simulink model "PruebaSupervisoryLogic"  (R2022a)
settings: Solver=VariableStepAuto  StartTime=0.0  StopTime=100  RelTol=1e-3
values from neighbouring files (symbols this model uses):
  a = 0.2    [Data.m]
  alturaobst = 0.9    [Data.m]
  b = 0.542    [Data.m]
  M = [x_new y_new]    [Data.m]
  M_chasis = 3.5    [Data.m]
  M_rueda = 1    [Data.m]
  M_ruedacontacto = 1    [Data.m]
  N = 4365    [GraficasVelocidades.m]    (also in Prueba_Liapunov.m = length(p_X); WaypointsToTrayectory.m = length(X))
  R = 0.175/2    (= 0.0875)    [Data.m]
  X = M(:,1)    [WaypointsToTrayectory.m]
  x0 = x_ini(1)*factorE    [Data.m]
  x_obj = pos_fin(1)*factorE    [Data.m]
  xobstac = RandomPos(1)    [Data.m]
  Y = M(:, 2)    [WaypointsToTrayectory.m]
  y0 = y_ini(2)*factorE    [Data.m]
  y_obj = pos_fin(2)*factorE    [Data.m]
  yobstac = RandomPos(2)    [Data.m]
  zobstac = RandomPos(3)    [Data.m]
undefined symbols (not defined in the file or in its folder): bloqueobstaculo, Borde11, Borde12, Borde2, Borde3, Borde41, Borde42, Explanada, plano150g1, plano150g2, plano150g3, plano150g4, Plano150mm, plano150mm2irr, Plano45mm, plano45mm2irr, Plano90mm, Rampa, Rampa21, Rampa22, Rampa31, Rampa32, Rampa33, Rampa4, Rampa51, Rampa52, Rampa53, Terreno, Z
libraries: sm_lib x331, nesl_utility x30, fl_lib x3, robotalgslib x1
(part 2 of 8)

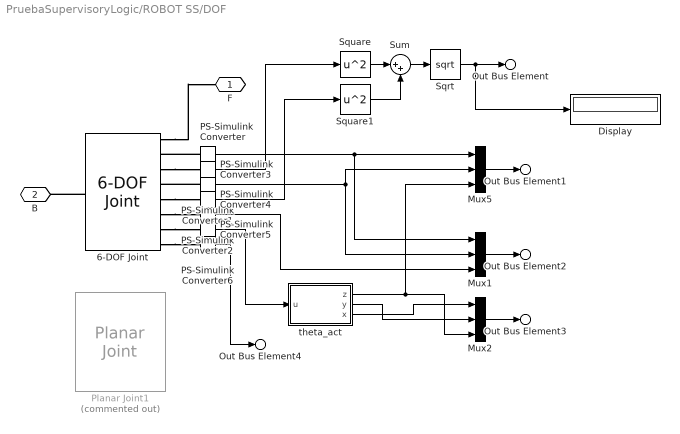
== system PruebaSupervisoryLogic/ROBOT SS/DOF ==
  6-DOF Joint : sm_lib/Joints/6-DOF Joint  JointMode=Normal  SenseConstraintForce=off  SenseConstraintForceX=off  SenseConstraintForceY=off  SenseConstraintForceZ=off  SenseConstraintTorque=off  SenseConstraintTorqueX=off  SenseConstraintTorqueY=off  SenseConstraintTorqueZ=off  SenseTotalForce=off  SenseTotalForceX=off  SenseTotalForceY=off  SenseTotalForceZ=off  SenseTotalTorque=off  SenseTotalTorqueX=off  SenseTotalTorqueY=off  SenseTotalTorqueZ=off  CompositeWrenchDir=FollowerOnBase  CompositeWrenchFrame=BaseFrame  PxEquilibriumPosition=0  PxEquilibriumPositionUnits=m  PxSpringStiffness=0  PxSpringStiffnessUnits=N/m  PxDampingCoefficient=0  PxDampingCoefficientUnits=N/(m/s)  PxTorqueActuationMode=NoTorque  PxMotionActuationMode=ComputedMotion  PxSensePosition=on  PxSenseVelocity=on  PxSenseAcceleration=off  PxSenseTorqueForce=off  PxSenseLowerLimitTorqueForce=off  PxSenseUpperLimitTorqueForce=off  PxLowerLimitSpecify=off  PxLowerLimitBound=-1  PxLowerLimitBoundUnits=m  PxLowerLimitStiffness=1e6  PxLowerLimitStiffnessUnits=N/m  PxLowerLimitDamping=1e3  PxLowerLimitDampingUnits=N/(m/s)  PxLowerLimitTransitionRegionWidth=1e-4  PxLowerLimitTransitionRegionWidthUnits=m  PxUpperLimitSpecify=off  PxUpperLimitBound=1  PxUpperLimitBoundUnits=m  PxUpperLimitStiffness=1e6  PxUpperLimitStiffnessUnits=N/m  PxUpperLimitDamping=1e3  PxUpperLimitDampingUnits=N/(m/s)  PxUpperLimitTransitionRegionWidth=1e-4  PxUpperLimitTransitionRegionWidthUnits=m  PxPositionTargetSpecify=on  PxPositionTargetPriority=High  PxPositionTargetValue=x0  PxPositionTargetValueUnits=m  PxVelocityTargetSpecify=off  PxVelocityTargetPriority=High  PxVelocityTargetValue=0  PxVelocityTargetValueUnits=m/s  PyEquilibriumPosition=0  PyEquilibriumPositionUnits=m  PySpringStiffness=0  PySpringStiffnessUnits=N/m  PyDampingCoefficient=0  PyDampingCoefficientUnits=N/(m/s)  PyTorqueActuationMode=NoTorque  PyMotionActuationMode=ComputedMotion  PySensePosition=on  PySenseVelocity=on  PySenseAcceleration=off  PySenseTorqueForce=off  PySenseLowerLimitTorqueForce=off  PySenseUpperLimitTorqueForce=off  PyLowerLimitSpecify=off  PyLowerLimitBound=-1  PyLowerLimitBoundUnits=m  PyLowerLimitStiffness=1e6  PyLowerLimitStiffnessUnits=N/m  PyLowerLimitDamping=1e3  PyLowerLimitDampingUnits=N/(m/s)  PyLowerLimitTransitionRegionWidth=1e-4  PyLowerLimitTransitionRegionWidthUnits=m  PyUpperLimitSpecify=off  PyUpperLimitBound=1  PyUpperLimitBoundUnits=m  PyUpperLimitStiffness=1e6  PyUpperLimitStiffnessUnits=N/m  PyUpperLimitDamping=1e3  PyUpperLimitDampingUnits=N/(m/s)  PyUpperLimitTransitionRegionWidth=1e-4  PyUpperLimitTransitionRegionWidthUnits=m  PyPositionTargetSpecify=on  PyPositionTargetPriority=High  PyPositionTargetValue=y0  PyPositionTargetValueUnits=m  PyVelocityTargetSpecify=off  PyVelocityTargetPriority=High  PyVelocityTargetValue=0  PyVelocityTargetValueUnits=m/s  PzEquilibriumPosition=0  PzEquilibriumPositionUnits=m  PzSpringStiffness=0  PzSpringStiffnessUnits=N/m  PzDampingCoefficient=0  PzDampingCoefficientUnits=N/(m/s)  PzTorqueActuationMode=NoTorque  PzMotionActuationMode=ComputedMotion  PzSensePosition=on  PzSenseVelocity=off  PzSenseAcceleration=off  PzSenseTorqueForce=off  PzSenseLowerLimitTorqueForce=off  PzSenseUpperLimitTorqueForce=off  PzLowerLimitSpecify=off  PzLowerLimitBound=-1  PzLowerLimitBoundUnits=m  PzLowerLimitStiffness=1e6  PzLowerLimitStiffnessUnits=N/m  PzLowerLimitDamping=1e3  PzLowerLimitDampingUnits=N/(m/s)  PzLowerLimitTransitionRegionWidth=1e-4  PzLowerLimitTransitionRegionWidthUnits=m  PzUpperLimitSpecify=off  PzUpperLimitBound=1  PzUpperLimitBoundUnits=m  PzUpperLimitStiffness=1e6  PzUpperLimitStiffnessUnits=N/m  PzUpperLimitDamping=1e3  PzUpperLimitDampingUnits=N/(m/s)  PzUpperLimitTransitionRegionWidth=1e-4  PzUpperLimitTransitionRegionWidthUnits=m  PzPositionTargetSpecify=off  PzPositionTargetPriority=High  PzPositionTargetValue=1  PzPositionTargetValueUnits=m  PzVelocityTargetSpecify=off  PzVelocityTargetPriority=High  PzVelocityTargetValue=0  PzVelocityTargetValueUnits=m/s  SphDefPosRotationMethod=None  SphDefPosRotationAngleUnits=deg  SphDefPosRotationStandardAxis=+Z  SphDefPosRotationAngle=0.0  SphDefPosRotationArbitraryAxis=[0 0 1]  SphDefPosFollAlignAxisA=+X  SphDefPosBaseAlignAxisA=+Y  SphDefPosFollAlignAxisB=+Y  SphDefPosBaseAlignAxisB=+Z  SphDefPosRotationSequenceAxes=FollowerAxes  SphDefPosRotationSequence=XYX  SphDefPosRotationSequenceAngles=[0 0 0]  SphDefPosRotationSequenceAnglesUnits=deg  SphDefPosRotationMatrix=[1 0 0; 0 1 0; 0 0 1]  SphEqPosRotationMethod=None  SphEqPosRotationAngleUnits=deg  SphEqPosRotationStandardAxis=+Z  SphEqPosRotationAngle=0.0  SphEqPosRotationArbitraryAxis=[0 0 1]  SphEqPosFollAlignAxisA=+X  SphEqPosBaseAlignAxisA=+Y  SphEqPosFollAlignAxisB=+Y  SphEqPosBaseAlignAxisB=+Z  SphEqPosRotationSequenceAxes=FollowerAxes  SphEqPosRotationSequence=XYX  SphEqPosRotationSequenceAngles=[0 0 0]  SphEqPosRotationSequenceAnglesUnits=deg  SphEqPosRotationMatrix=[1 0 0; 0 1 0; 0 0 1]  SphSpringStiffness=0  SphSpringStiffnessUnits=N*m/deg  SphDampingCoefficient=0  SphDampingCoefficientUnits=N*m/(deg/s)  SphActuateTorqueX=off  SphActuateTorqueY=off  SphActuateTorqueZ=off  SphActuateTorque=off  SphTorqueActuationMode=NoTorque  SphMotionActuationMode=ComputedMotion  SphActuationFrame=BaseFrame  SphSensePosition=on  SphSenseVelocityX=off  SphSenseVelocityY=off  SphSenseVelocityZ=on  SphSenseVelocity=off  SphSenseAccelerationX=off  SphSenseAccelerationY=off  SphSenseAccelerationZ=off  SphSenseAcceleration=off  SphSenseTorqueX=off  SphSenseTorqueY=off  SphSenseTorqueZ=off  SphSenseTorqueForce=off  SphSenseLowerLimitTorqueMag=off  SphSenseUpperLimitTorqueMag=off  SphSensingFrame=BaseFrame  SphLowerLimitSpecify=off  SphLowerLimitBound=15  SphLowerLimitBoundUnits=deg  SphLowerLimitStiffness=1e4  SphLowerLimitStiffnessUnits=N*m/deg  SphLowerLimitDamping=10  SphLowerLimitDampingUnits=N*m/(deg/s)  SphLowerLimitTransitionRegionWidth=0.1  SphLowerLimitTransitionRegionWidthUnits=deg  SphUpperLimitSpecify=off  SphUpperLimitBound=45  SphUpperLimitBoundUnits=deg  SphUpperLimitStiffness=1e4  SphUpperLimitStiffnessUnits=N*m/deg  SphUpperLimitDamping=10  SphUpperLimitDampingUnits=N*m/(deg/s)  SphUpperLimitTransitionRegionWidth=0.1  SphUpperLimitTransitionRegionWidthUnits=deg  SphPositionTargetRotationMethod=StandardAxis  SphPositionTargetRotationAngleUnits=rad  SphPositionTargetRotationStandardAxis=+Z  SphPositionTargetRotationAngle=2*pi  SphPositionTargetRotationArbitraryAxis=[0 0 1]  SphPositionTargetFollAlignAxisA=+X  SphPositionTargetBaseAlignAxisA=+Y  SphPositionTargetFollAlignAxisB=+Y  SphPositionTargetBaseAlignAxisB=+Z  SphPositionTargetRotationSequenceAxes=FollowerAxes  SphPositionTargetRotationSequence=ZYX  SphPositionTargetRotationSequenceAngles=[0.0532 -0.048 0.0147]  SphPositionTargetRotationSequenceAnglesUnits=rad  SphPositionTargetRotationMatrix=[1 0 0; 0 1 0; 0 0 1]  SphPositionTargetSpecify=on  SphPositionTargetPriority=High  SphVelocityTargetValue=[0 0 0]  SphVelocityTargetValueUnits=deg/s  SphVelocityTargetSpecify=off  SphVelocityTargetPriority=High  SphVelocityTargetInFollowerFrame=on
  Display : Display
  Mux1 : Mux  Inputs=3
  Mux2 : Mux  Inputs=3
  Mux5 : Mux  Inputs=3
  PS-Simulink Converter{,1..6} (7 alike) : nesl_utility/PS-Simulink Converter  PhysicalDomain=network_engine_domain  SubClassName=ps_output  LeftPortType=input  RightPortType=output  PseudoPeriodic=off  Frequencies=[]  VectorFormat=inherit  Unit=inherit  AffineConversion=off
      settings: SourceProductBaseCode=SS,PW,VE
  Planar Joint1 : sm_lib/Joints/Planar Joint  Commented=on  JointMode=Normal  SenseConstraintForce=off  SenseConstraintForceX=off  SenseConstraintForceY=off  SenseConstraintForceZ=off  SenseConstraintTorque=off  SenseConstraintTorqueX=off  SenseConstraintTorqueY=off  SenseConstraintTorqueZ=off  SenseTotalForce=off  SenseTotalForceX=off  SenseTotalForceY=off  SenseTotalForceZ=off  SenseTotalTorque=off  SenseTotalTorqueX=off  SenseTotalTorqueY=off  SenseTotalTorqueZ=off  CompositeWrenchDir=FollowerOnBase  CompositeWrenchFrame=BaseFrame  PxEquilibriumPosition=0  PxEquilibriumPositionUnits=m  PxSpringStiffness=0  PxSpringStiffnessUnits=N/m  PxDampingCoefficient=0  PxDampingCoefficientUnits=N/(m/s)  PxTorqueActuationMode=NoTorque  PxMotionActuationMode=ComputedMotion  PxSensePosition=on  PxSenseVelocity=off  PxSenseAcceleration=off  PxSenseTorqueForce=off  PxSenseLowerLimitTorqueForce=off  PxSenseUpperLimitTorqueForce=off  PxLowerLimitSpecify=off  PxLowerLimitBound=-1  PxLowerLimitBoundUnits=m  PxLowerLimitStiffness=1e6  PxLowerLimitStiffnessUnits=N/m  PxLowerLimitDamping=1e3  PxLowerLimitDampingUnits=N/(m/s)  PxLowerLimitTransitionRegionWidth=1e-4  PxLowerLimitTransitionRegionWidthUnits=m  PxUpperLimitSpecify=off  PxUpperLimitBound=1  PxUpperLimitBoundUnits=m  PxUpperLimitStiffness=1e6  PxUpperLimitStiffnessUnits=N/m  PxUpperLimitDamping=1e3  PxUpperLimitDampingUnits=N/(m/s)  PxUpperLimitTransitionRegionWidth=1e-4  PxUpperLimitTransitionRegionWidthUnits=m  PxPositionTargetSpecify=on  PxPositionTargetPriority=High  PxPositionTargetValue=540  PxPositionTargetValueUnits=m  PxVelocityTargetSpecify=off  PxVelocityTargetPriority=High  PxVelocityTargetValue=0  PxVelocityTargetValueUnits=m/s  PyEquilibriumPosition=0  PyEquilibriumPositionUnits=m  PySpringStiffness=0  PySpringStiffnessUnits=N/m  PyDampingCoefficient=0  PyDampingCoefficientUnits=N/(m/s)  PyTorqueActuationMode=NoTorque  PyMotionActuationMode=ComputedMotion  PySensePosition=on  PySenseVelocity=off  PySenseAcceleration=off  PySenseTorqueForce=off  PySenseLowerLimitTorqueForce=off  PySenseUpperLimitTorqueForce=off  PyLowerLimitSpecify=off  PyLowerLimitBound=-1  PyLowerLimitBoundUnits=m  PyLowerLimitStiffness=1e6  PyLowerLimitStiffnessUnits=N/m  PyLowerLimitDamping=1e3  PyLowerLimitDampingUnits=N/(m/s)  PyLowerLimitTransitionRegionWidth=1e-4  PyLowerLimitTransitionRegionWidthUnits=m  PyUpperLimitSpecify=off  PyUpperLimitBound=1  PyUpperLimitBoundUnits=m  PyUpperLimitStiffness=1e6  PyUpperLimitStiffnessUnits=N/m  PyUpperLimitDamping=1e3  PyUpperLimitDampingUnits=N/(m/s)  PyUpperLimitTransitionRegionWidth=1e-4  PyUpperLimitTransitionRegionWidthUnits=m  PyPositionTargetSpecify=on  PyPositionTargetPriority=High  PyPositionTargetValue=241  PyPositionTargetValueUnits=m  PyVelocityTargetSpecify=off  PyVelocityTargetPriority=High  PyVelocityTargetValue=0  PyVelocityTargetValueUnits=m/s  RzEquilibriumPosition=0  RzEquilibriumPositionUnits=deg  RzSpringStiffness=0  RzSpringStiffnessUnits=N*m/deg  RzDampingCoefficient=0  RzDampingCoefficientUnits=N*m/(deg/s)  RzTorqueActuationMode=NoTorque  RzMotionActuationMode=ComputedMotion  RzSensePosition=on  RzSenseVelocity=off  RzSenseAcceleration=off  RzSenseTorqueForce=off  RzSenseLowerLimitTorqueForce=off  RzSenseUpperLimitTorqueForce=off  RzLowerLimitSpecify=off  RzLowerLimitBound=-90  RzLowerLimitBoundUnits=deg  RzLowerLimitStiffness=1e4  RzLowerLimitStiffnessUnits=N*m/deg  RzLowerLimitDamping=10  RzLowerLimitDampingUnits=N*m/(deg/s)  RzLowerLimitTransitionRegionWidth=0.1  RzLowerLimitTransitionRegionWidthUnits=deg  RzUpperLimitSpecify=off  RzUpperLimitBound=90  RzUpperLimitBoundUnits=deg  RzUpperLimitStiffness=1e4  RzUpperLimitStiffnessUnits=N*m/deg  RzUpperLimitDamping=10  RzUpperLimitDampingUnits=N*m/(deg/s)  RzUpperLimitTransitionRegionWidth=0.1  RzUpperLimitTransitionRegionWidthUnits=deg  RzPositionTargetSpecify=on  RzPositionTargetPriority=High  RzPositionTargetValue=2*pi/3  RzPositionTargetValueUnits=rad  RzVelocityTargetSpecify=off  RzVelocityTargetPriority=High  RzVelocityTargetValue=0  RzVelocityTargetValueUnits=deg/s
  Sqrt : Sqrt
  Square : Math  Operator=square
  Square1 : Math  Operator=square
  Sum : Sum  Inputs=|++
  theta_act : MATLAB Function  TreatAsAtomicUnit=on
  F : PMIOPort  Side=Right
  B : PMIOPort  Port=2  Side=Left
  Out Bus Element : Outport  PortName=dof  Element=v
  Out Bus Element1 : Outport  PortName=dof  Element=Pose
  Out Bus Element2 : Outport  PortName=dof  Element=xyz
  Out Bus Element3 : Outport  PortName=dof  Element=rpy
  Out Bus Element4 : Outport  PortName=dof  Element=wz
  wires:
  PS-Simulink Converter/1 -> Mux1/1, Mux5/1
  Mux5/1 -> Out Bus Element1/1
  PS-Simulink Converter1/1 -> Mux1/2, Mux5/2
  Square1/1 -> Sum/2
  PS-Simulink Converter4/1 -> Square1/1
  Sum/1 -> Sqrt/1
  Square/1 -> Sum/1
  PS-Simulink Converter3/1 -> Square/1
  Sqrt/1 -> Display/1, Out Bus Element/1
  PS-Simulink Converter2/1 -> Mux1/3
  Mux1/1 -> Out Bus Element2/1
  PS-Simulink Converter5/1 -> theta_act/1(u)
  theta_act/1(z) -> Mux5/3, Mux2/3
  theta_act/3(x) -> Mux2/1
  theta_act/2(y) -> Mux2/2
  Mux2/1 -> Out Bus Element3/1
  PS-Simulink Converter6/1 -> Out Bus Element4/1
  connections:
  PS-Simulink Converter/LConn1 -- 6-DOF Joint/RConn2
  6-DOF Joint/LConn1 -- B/RConn1
  PS-Simulink Converter1/LConn1 -- 6-DOF Joint/RConn4
  6-DOF Joint/RConn1 -- F/RConn1
  6-DOF Joint/RConn3 -- PS-Simulink Converter3/LConn1
  6-DOF Joint/RConn5 -- PS-Simulink Converter4/LConn1
  6-DOF Joint/RConn6 -- PS-Simulink Converter2/LConn1
  6-DOF Joint/RConn7 -- PS-Simulink Converter5/LConn1
  6-DOF Joint/RConn8 -- PS-Simulink Converter6/LConn1

== system PruebaSupervisoryLogic/ROBOT SS/DesPathViz ==
  Desired Path Viz : sm_lib/Curves and Surfaces/Point Cloud  CoordinatesMatrix=pointCloud  CoordinatesMatrixUnits=m  GraphicType=MarkerCloud  GraphicSphereRadius=0.03  GraphicSphereRadiusUnits=m  GraphicVisPropType=SimpleVisualProperties  GraphicDiffuseColor=[0 0 1]  GraphicOpacity=1  GraphicSpecularColor=[0.5 0.5 0.5 1.0]  GraphicAmbientColor=[0.15 0.15 0.15 1.0]  GraphicEmissiveColor=[0.0 0.0 0.0 1.0]  GraphicShininess=75
      settings: SourceProductBaseCode=MS
  Rigid Transform6 : sm_lib/Frames and Transforms/Rigid Transform  TranslationMethod=Cartesian  TranslationStandardOffset=1.85  TranslationLengthUnit=m  TranslationStandardAxis=+Z  TranslationCartesianOffset=[0 0 0]  TranslationROffset=0  TranslationROffsetUnits=m  TranslationZOffset=0  TranslationZOffsetUnits=m  TranslationThetaOffset=0  TranslationThetaOffsetUnits=deg  RotationMethod=None  RotationAngleUnits=deg  RotationStandardAxis=+X  RotationAngle=90  RotationArbitraryAxis=[0 0 1]  FollAlignAxisA=+X  BaseAlignAxisA=+Y  FollAlignAxisB=+Y  BaseAlignAxisB=+Z  RotationSequenceAxes=FollowerAxes  RotationSequence=XYX  RotationSequenceAngles=[0 0 0]  RotationSequenceAnglesUnits=deg  RotationMatrix=[1 0 0; 0 1 0; 0 0 1]
  Spline : sm_lib/Curves and Surfaces/Spline  GraphicAmbientColor=[0.15 0.15 0.15 1.0]  GraphicDiffuseColor=[0 0.4471 0.7412]  DataPoints=pointCloud  DataPointsUnits=m  GraphicEmissiveColor=[0.0 0.0 0.0 1.0]  EndConditionType=Natural  MarkerShape=Sphere  MarkerSize=10  GraphicType=FromGeometry  GraphicOpacity=1  GraphicShininess=75  GraphicSpecularColor=[0.5 0.5 0.5 1.0]  GraphicVisPropType=SimpleVisualProperties
  R : PMIOPort  Side=Left
  connections:
  R/RConn1 -- Rigid Transform6/LConn1
  Rigid Transform6/RConn1 -- Desired Path Viz/LConn1 -- Spline/LConn1

== system PruebaSupervisoryLogic/ROBOT SS/Ensamble robot ==
  In1 : Inport
  In2 : Inport  Port=2
  Chasis : Subsystem
      settings: PortSchema="{\"entries\":[{\"content\":{\"sides\":[{\"content\":{\"connectorIds\":[\"LConn1\",\"LConn2\"]},\"type\":\"ConnectorPlacement.EquallySpacedRectSide\",\"uuid\":\"70add61d-4d2b-4209-9064-ae93618a5dda\"},{\"content\":{\"connectorIds\":[\"RConn1\",\"RConn2\"],\"side\":\"RIGHT\"},\"type\":\"ConnectorPlacement.EquallySpacedRectSide\",\"uuid\":\"c0cb1301-4b60-4f09-9729-118a381e7d2b\"},{\"content\":{\"connectorIds\":[\"LConn3\",\"LConn4\"],\"side\":\"TOP\"},\"type\":\"ConnectorPlacement.EquallySpacedRectSide\",\"uuid\":\"bcc4c9f8-927c-42da-82df-989f649289ae\"},{\"content\":{\"connectorIds\":[\"RConn3\"],\"side\":\"BOTTOM\"},\"type\":\"ConnectorPlacement.EquallySpacedRectSide\",\"uuid\":\"275f36ca-265b-4208-becd-8d42af8e2e6a\"}]},\"type\":\"ConnectorPlacement.EquallySpacedConnector\",\"uuid\":\"a4bbac37-5f09-4c0c-9b07-eae0fbc73e5d\"}],\"packageUris\":[\"http://schema.mathworks.com/mf0/Connector/R2020b\"],\"version\":\"1.0\"}"
  ContactosRueas4 : Subsystem
  Integrator : Integrator
  Integrator1 : Integrator
  RDBack : Subsystem
  RDFront : Subsystem
  RIBack : Subsystem
      settings: PortSchema="{\"entries\":[{\"content\":{\"sides\":[{\"content\":{\"connectorIds\":[\"LConn1\",\"Out1\"]},\"type\":\"ConnectorPlacement.EquallySpacedRectSide\",\"uuid\":\"5939dff2-20e4-419e-9479-36ab2354c98a\"},{\"content\":{\"connectorIds\":[\"RConn1\"],\"side\":\"RIGHT\"},\"type\":\"ConnectorPlacement.EquallySpacedRectSide\",\"uuid\":\"e7e2d6de-4e85-41ae-b0fc-f1d38849587e\"},{\"content\":{\"connectorIds\":[],\"side\":\"TOP\"},\"type\":\"ConnectorPlacement.EquallySpacedRectSide\",\"uuid\":\"92513f77-6228-42a9-918c-62f3b48e4ee8\"},{\"content\":{\"connectorIds\":[\"RConn2\"],\"side\":\"BOTTOM\"},\"type\":\"ConnectorPlacement.EquallySpacedRectSide\",\"uuid\":\"7a57670a-e20e-4db3-92b5-cb403023e5be\"}]},\"type\":\"ConnectorPlacement.EquallySpacedConnector\",\"uuid\":\"ca332874-eec6-4d24-915b-f15236e30e05\"}],\"packageUris\":[\"http://schema.mathworks.com/mf0/Connector/R2020b\"],\"version\":\"1.0\"}"
  RIFront : Subsystem
      settings: PortSchema="{\"entries\":[{\"content\":{\"sides\":[{\"content\":{\"connectorIds\":[\"LConn1\",\"Out1\"]},\"type\":\"ConnectorPlacement.EquallySpacedRectSide\",\"uuid\":\"1a6d18f2-9060-460a-a6d5-9e4b3eb03e79\"},{\"content\":{\"connectorIds\":[\"RConn1\"],\"side\":\"RIGHT\"},\"type\":\"ConnectorPlacement.EquallySpacedRectSide\",\"uuid\":\"17ea15c1-ecd0-4eab-a22a-1bc805986bcc\"},{\"content\":{\"connectorIds\":[],\"side\":\"TOP\"},\"type\":\"ConnectorPlacement.EquallySpacedRectSide\",\"uuid\":\"77550975-b499-4629-bedd-c387e5873676\"},{\"content\":{\"connectorIds\":[\"RConn2\"],\"side\":\"BOTTOM\"},\"type\":\"ConnectorPlacement.EquallySpacedRectSide\",\"uuid\":\"13653250-c8e4-4613-b3da-0c20385c9486\"}]},\"type\":\"ConnectorPlacement.EquallySpacedConnector\",\"uuid\":\"3bb9ea0c-1132-4bf2-af47-0db6481cd1ef\"}],\"packageUris\":[\"http://schema.mathworks.com/mf0/Connector/R2020b\"],\"version\":\"1.0\"}"
  Simscape Bus : SimscapeBus  HierarchyStrings=plano150mm2irr;plano45mm2irr;bloqueobstaculo;Borde42;Borde41;Borde3;Borde2;Borde12;Borde11;Plano150mm;Plano90mm;Plano45mm;Terreno;Rampa;Explanada
  Simscape Bus1 : SimscapeBus  HierarchyStrings=plano150g4;plano150g3;plano150g2;plano150g1;Rampa21;Rampa22;Rampa31;Rampa32;Rampa33;Rampa4;Rampa51;Rampa52;Rampa53
  Simulink-PS Converter{1..2,4..5} (4 alike) : nesl_utility/Simulink-PS Converter  PhysicalDomain=network_engine_domain  SubClassName=ps_input  LeftPortType=input  RightPortType=output  PseudoPeriodic=off  Frequencies=[]  NoiseDistribution=none  NoiseParameters=[]  Unit=1  AffineConversion=off  FilteringAndDerivatives=filter  SimscapeFilterOrder=2  InputFilterTimeConstant=0.001  UdotUserProvided=0
      settings: SourceProductBaseCode=SS,PW,VE
  Tapa : Subsystem
  Transform Floor : sm_lib/Frames and Transforms/Rigid Transform  TranslationMethod=StandardAxis  TranslationStandardOffset=-5.75  TranslationLengthUnit=cm  TranslationStandardAxis=+Z  TranslationCartesianOffset=[0 0 0]  TranslationROffset=0  TranslationROffsetUnits=m  TranslationZOffset=0  TranslationZOffsetUnits=m  TranslationThetaOffset=0  TranslationThetaOffsetUnits=deg  RotationMethod=StandardAxis  RotationAngleUnits=deg  RotationStandardAxis=+Z  RotationAngle=0*15  RotationArbitraryAxis=[0 0 1]  FollAlignAxisA=+X  BaseAlignAxisA=+Y  FollAlignAxisB=+Y  BaseAlignAxisB=+Z  RotationSequenceAxes=FollowerAxes  RotationSequence=XYX  RotationSequenceAngles=[0 0 0]  RotationSequenceAnglesUnits=deg  RotationMatrix=[1 0 0; 0 1 0; 0 0 1]
  F : PMIOPort  Side=Right
  ContactZ : PMIOPort  Port=2  Side=Left
  tag scope: w1act=global, w2act=global, w3act=global, w4act=global
  wires:
  In1/1 -> Integrator/1
  Integrator/1 -> Simulink-PS Converter5/1, Simulink-PS Converter4/1
  Integrator1/1 -> Simulink-PS Converter1/1, Simulink-PS Converter2/1
  RIFront/1(ws) -> [w3act]
  RDBack/1(ws) -> [w2act]
  RDFront/1(ws) -> [w1act]
  RIBack/1(ws) -> [w4act]
  In2/1 -> Integrator1/1
  connections:
  Chasis/RConn3 -- Transform Floor/LConn1
  RIFront/LConn1 -- Simulink-PS Converter2/RConn1
  Tapa/LConn1 -- Chasis/LConn3
  RIFront/RConn1 -- Chasis/RConn1
  Simulink-PS Converter5/RConn1 -- RDBack/LConn1
  F/RConn1 -- Transform Floor/RConn1
  Chasis/LConn1 -- RDFront/RConn1
  RIBack/RConn1 -- Chasis/RConn2
  Simulink-PS Converter4/RConn1 -- RDFront/LConn1
  ContactZ/RConn1 -- Simscape Bus/RConn1 -- Simscape Bus1/RConn1
  RDBack/RConn1 -- Chasis/LConn2
  Simulink-PS Converter1/RConn1 -- RIBack/LConn1
  ContactosRueas4/RConn1 -- RDFront/LConn2
  ContactosRueas4/RConn2 -- RDBack/LConn2
  RIFront/RConn2 -- ContactosRueas4/RConn3
  ContactosRueas4/RConn4 -- RIBack/RConn2
  Simscape Bus/LConn14 -- ContactosRueas4/LConn14
  ContactosRueas4/LConn12 -- Simscape Bus/LConn12
  ContactosRueas4/LConn11 -- Simscape Bus/LConn11
  ContactosRueas4/LConn10 -- Simscape Bus/LConn10
  ContactosRueas4/LConn15 -- Simscape Bus/LConn15
  ContactosRueas4/LConn13 -- Simscape Bus/LConn13
  Simscape Bus1/LConn5 -- ContactosRueas4/LConn20
  Simscape Bus1/LConn6 -- ContactosRueas4/LConn21
  Simscape Bus/LConn5 -- ContactosRueas4/LConn5
  Simscape Bus/LConn6 -- ContactosRueas4/LConn6
  Simscape Bus/LConn7 -- ContactosRueas4/LConn7
  Simscape Bus/LConn8 -- ContactosRueas4/LConn8
  Simscape Bus/LConn9 -- ContactosRueas4/LConn9
  Chasis/LConn4 -- ContactosRueas4/RConn5
  Simscape Bus/LConn4 -- ContactosRueas4/LConn4
  Simscape Bus/LConn1 -- ContactosRueas4/LConn1
  Simscape Bus/LConn2 -- ContactosRueas4/LConn2
  Simscape Bus/LConn3 -- ContactosRueas4/LConn3
  Simscape Bus1/LConn1 -- ContactosRueas4/LConn16
  Simscape Bus1/LConn2 -- ContactosRueas4/LConn17
  Simscape Bus1/LConn3 -- ContactosRueas4/LConn18
  Simscape Bus1/LConn4 -- ContactosRueas4/LConn19
  Simscape Bus1/LConn7 -- ContactosRueas4/LConn22
  Simscape Bus1/LConn8 -- ContactosRueas4/LConn23
  ContactosRueas4/LConn24 -- Simscape Bus1/LConn9
  ContactosRueas4/LConn25 -- Simscape Bus1/LConn10
  ContactosRueas4/LConn28 -- Simscape Bus1/LConn13
  ContactosRueas4/LConn26 -- Simscape Bus1/LConn11
  Simscape Bus1/LConn12 -- ContactosRueas4/LConn27

== system PruebaSupervisoryLogic/ROBOT SS/Subsystem ==
  Mux : Mux  Inputs=3
  PS-Simulink Converter{1..5,8} (6 alike) : nesl_utility/PS-Simulink Converter  PhysicalDomain=network_engine_domain  SubClassName=ps_output  LeftPortType=input  RightPortType=output  PseudoPeriodic=off  Frequencies=[]  VectorFormat=inherit  Unit=inherit  AffineConversion=off
      settings: SourceProductBaseCode=SS,PW,VE
  Rot 2 eul : MATLAB Function  TreatAsAtomicUnit=on
  Scope : Scope
  Transform Sensor : sm_lib/Frames and Transforms/Transform Sensor  MeasurementFrame=Base  SenseAngle=off  SenseAxis=off  SenseAngle1=off  SenseAngle2=off  SenseAngle3=off  SenseQ=off  SenseR=on  SenseOmegaX=off  SenseOmegaY=off  SenseOmegaZ=off  SenseOmega1=off  SenseOmega2=off  SenseOmega3=off  SenseQDot=off  SenseRDot=off  SenseAlphaX=off  SenseAlphaY=off  SenseAlphaZ=off  SenseAlpha1=off  SenseAlpha2=off  SenseAlpha3=off  SenseQDDot=off  SenseRDDot=off  SenseX=on  SenseY=on  SenseZ=on  SenseRad=off  SenseAzim=off  SenseDist=off  SenseInc=off  SenseXDot=on  SenseYDot=on  SenseZDot=off  SenseRadDot=off  SenseAzimDot=off  SenseDistDot=off  SenseIncDot=off  SenseXDDot=off  SenseYDDot=off  SenseZDDot=off  SenseRadDDot=off  SenseAzimDDot=off  SenseDistDDot=off  SenseIncDDot=off
  Vlineal : MATLAB Function  TreatAsAtomicUnit=on
  B : PMIOPort  Side=Left
  F : PMIOPort  Port=2  Side=Right
  Pose : Outport
  vsens : Outport  Port=2
  wires:
  Rot 2 eul/1(z) -> Mux/3
  PS-Simulink Converter2/1 -> Rot 2 eul/1(R)
  Mux/1 -> Pose/1
  Vlineal/1(v) -> vsens/1
  PS-Simulink Converter8/1 -> Mux/1
  PS-Simulink Converter3/1 -> Mux/2
  PS-Simulink Converter4/1 -> Vlineal/1(vx)
  PS-Simulink Converter5/1 -> Vlineal/2(vy)
  PS-Simulink Converter1/1 -> Scope/1
  connections:
  Transform Sensor/RConn4 -- PS-Simulink Converter3/LConn1
  Transform Sensor/RConn2 -- PS-Simulink Converter2/LConn1
  PS-Simulink Converter8/LConn1 -- Transform Sensor/RConn3
  Transform Sensor/LConn1 -- B/RConn1
  Transform Sensor/RConn1 -- F/RConn1
  Transform Sensor/RConn6 -- PS-Simulink Converter4/LConn1
  Transform Sensor/RConn7 -- PS-Simulink Converter5/LConn1
  PS-Simulink Converter1/LConn1 -- Transform Sensor/RConn5

== system PruebaSupervisoryLogic/Sensores Frente x7/Percepción_Central ==
  R_Pose : Inport
  Gain : Gain  Gain=pi/180
  Gain1 : Gain  Gain=pi/180
  Gain2 : Gain  Gain=pi/180
  Phi_Sensor : Constant  Value=0
  Phi_Sensor1 : Constant  Value=-20
  Phi_Sensor2 : Constant  Value=20
  Pos Obstaculo : Constant  Value=[xobstac; yobstac]
  Pos Obstaculo1 : Constant  Value=[xobstac; yobstac]
  Pos Obstaculo2 : Constant  Value=[xobstac; yobstac]
  SensorUltrasonido : Subsystem
  SensorUltrasonido1 : Subsystem
  SensorUltrasonido2 : Subsystem
  d_sensor : Constant  Value=0.25
  d_sensor1 : Constant  Value=0.25
  d_sensor2 : Constant  Value=0.25
  d_3 : Outport
  d_4 : Outport  Port=2
  d_5 : Outport  Port=3
  wires:
  SensorUltrasonido2/1(d) -> d_3/1
  Gain1/1 -> SensorUltrasonido1/2(PhiSensor)
  d_sensor/1 -> SensorUltrasonido/3(di_sensor)
  d_sensor1/1 -> SensorUltrasonido1/3(di_sensor)
  Phi_Sensor2/1 -> Gain2/1
  Gain2/1 -> SensorUltrasonido2/2(PhiSensor)
  Phi_Sensor1/1 -> Gain1/1
  SensorUltrasonido1/1(d) -> d_5/1
  Pos Obstaculo1/1 -> SensorUltrasonido1/1(Obs_Pose)
  Pos Obstaculo2/1 -> SensorUltrasonido2/1(Obs_Pose)
  d_sensor2/1 -> SensorUltrasonido2/3(di_sensor)
  Phi_Sensor/1 -> Gain/1
  Pos Obstaculo/1 -> SensorUltrasonido/1(Obs_Pose)
  SensorUltrasonido/1(d) -> d_4/1
  Gain/1 -> SensorUltrasonido/2(PhiSensor)
  R_Pose/1 -> SensorUltrasonido2/4(R_Pose), SensorUltrasonido1/4(R_Pose), SensorUltrasonido/4(R_Pose)

== system PruebaSupervisoryLogic/Sensores Frente x7/Percepción_Derecha ==
  R_Pose : Inport
  Gain : Gain  Gain=pi/180
  Gain1 : Gain  Gain=pi/180
  Phi_Sensor : Constant  Value=-40
  Phi_Sensor1 : Constant  Value=-70
  Pos Obstaculo : Constant  Value=[xobstac; yobstac]
  Pos Obstaculo1 : Constant  Value=[xobstac; yobstac]
  SensorUltrasonido : Subsystem
  SensorUltrasonido1 : Subsystem
  d_sensor : Constant  Value=0.25
  d_sensor1 : Constant  Value=0.25
  d_6 : Outport
  d_7 : Outport  Port=2
  wires:
  Gain1/1 -> SensorUltrasonido1/2(PhiSensor)
  d_sensor/1 -> SensorUltrasonido/3(di_sensor)
  d_sensor1/1 -> SensorUltrasonido1/3(di_sensor)
  Phi_Sensor1/1 -> Gain1/1
  SensorUltrasonido1/1(d) -> d_7/1
  Pos Obstaculo1/1 -> SensorUltrasonido1/1(Obs_Pose)
  Phi_Sensor/1 -> Gain/1
  Pos Obstaculo/1 -> SensorUltrasonido/1(Obs_Pose)
  SensorUltrasonido/1(d) -> d_6/1
  Gain/1 -> SensorUltrasonido/2(PhiSensor)
  R_Pose/1 -> SensorUltrasonido1/4(R_Pose), SensorUltrasonido/4(R_Pose)

== system PruebaSupervisoryLogic/Sensores Frente x7/Percepción_Izquierda ==
  R_Pose : Inport
  Gain : Gain  Gain=pi/180
  Gain1 : Gain  Gain=pi/180
  Phi_Sensor : Constant  Value=70
  Phi_Sensor1 : Constant  Value=40
  Pos Obstaculo : Constant  Value=[xobstac; yobstac]
  Pos Obstaculo1 : Constant  Value=[xobstac; yobstac]
  SensorUltrasonido : Subsystem
  SensorUltrasonido1 : Subsystem
  d_sensor : Constant  Value=0.25
  d_sensor1 : Constant  Value=0.25
  d_1 : Outport
  d_2 : Outport  Port=2
  wires:
  R_Pose/1 -> SensorUltrasonido/4(R_Pose), SensorUltrasonido1/4(R_Pose)
  Gain/1 -> SensorUltrasonido/2(PhiSensor)
  SensorUltrasonido/1(d) -> d_1/1
  Pos Obstaculo/1 -> SensorUltrasonido/1(Obs_Pose)
  Phi_Sensor/1 -> Gain/1
  Pos Obstaculo1/1 -> SensorUltrasonido1/1(Obs_Pose)
  SensorUltrasonido1/1(d) -> d_2/1
  Phi_Sensor1/1 -> Gain1/1
  d_sensor1/1 -> SensorUltrasonido1/3(di_sensor)
  d_sensor/1 -> SensorUltrasonido/3(di_sensor)
  Gain1/1 -> SensorUltrasonido1/2(PhiSensor)

== system PruebaSupervisoryLogic/Path Planning1/Kinematics1/Inverse-Kinematics ==
  v : Inport
  w : Inport  Port=2
  Gain : Gain  Gain=b/2
  Gain1 : Gain  Gain=1/R
  Gain2 : Gain  Gain=1/R
  Sum : Sum  Inputs=|+-
  Sum1 : Sum  Inputs=|++
  wL : Outport
  wR : Outport  Port=2
  wires:
  w/1 -> Gain/1
  Sum1/1 -> Gain2/1
  v/1 -> Sum/1, Sum1/1
  Gain2/1 -> wR/1
  Gain1/1 -> wL/1
  Sum/1 -> Gain1/1
  Gain/1 -> Sum/2, Sum1/2

== system PruebaSupervisoryLogic/Path Planning2/Kinematics1/Direct-Kinematics ==
  wl : Inport
  wr : Inport  Port=2
  w : Inport  Port=3
  Constant : Constant  Value=[540 241 2*pi/3]
  Constant1 : Constant  Value=0.08
  Constant2 : Constant  Value=2*a
  Constant3 : Constant  Value=b
  Integrator2 : Integrator
  Integrator3 : Integrator  InitialCondition=x0
  Integrator4 : Integrator  InitialCondition=y0
  MATLAB Function : MATLAB Function  TreatAsAtomicUnit=on
  Mux : Mux  Inputs=3
  Pose : Outport
  wires:
  Mux/1 -> Pose/1
  Integrator4/1 -> Mux/2
  Constant3/1 -> MATLAB Function/5(a)
  MATLAB Function/3(o) -> Mux/3
  MATLAB Function/1(xp) -> Integrator3/1
  Integrator3/1 -> Mux/1
  Integrator2/1 -> MATLAB Function/6(or)
  w/1 -> Integrator2/1
  wr/1 -> MATLAB Function/1(wr)
  Constant1/1 -> MATLAB Function/3(r)
  MATLAB Function/2(yp) -> Integrator4/1
  Constant2/1 -> MATLAB Function/4(c)
  wl/1 -> MATLAB Function/2(wl)

== system PruebaSupervisoryLogic/Path Planning2/Kinematics1/Inverse-Kinematics ==
  v : Inport
  w : Inport  Port=2
  Gain : Gain  Gain=b/2
  Gain1 : Gain  Gain=1/R
  Gain2 : Gain  Gain=1/R
  Sum : Sum  Inputs=|+-
  Sum1 : Sum  Inputs=|++
  wL : Outport
  wR : Outport  Port=2
  wires:
  Gain/1 -> Sum1/2, Sum/2
  Sum/1 -> Gain1/1
  Gain1/1 -> wL/1
  Gain2/1 -> wR/1
  v/1 -> Sum1/1, Sum/1
  Sum1/1 -> Gain2/1
  w/1 -> Gain/1

== system PruebaSupervisoryLogic/Path Planning2/Subsystem1/check-goal ==
  Pose : Inport
  Constant : Constant  Value=[x_obj ,y_obj]
  MATLAB Function : MATLAB Function  TreatAsAtomicUnit=on
  Scope : Scope
  Selector : Selector  InputPortWidth=3  IndexOptions=Index vector (dialog)  Indices=[1 2]  OutputSizes=1
  distanceGoal : Outport
  wires:
  MATLAB Function/1(distanceGoal) -> Scope/1, distanceGoal/1
  Constant/1 -> MATLAB Function/2(goal)
  Selector/1 -> MATLAB Function/1(posexy)
  Pose/1 -> Selector/1

== system PruebaSupervisoryLogic/Path Planning2/hold/StopTime ==
  Enable : Inport
  Clock : Clock
  Constant2 : Constant
  Display : Display
  Enabled Subsystem1 : Subsystem  TreatAsAtomicUnit=on
      settings: MinAlgLoopOccurrences=on
  Switch : Switch  Criteria=u2 > Threshold  SaturateOnIntegerOverflow=off  InputSameDT=off
  Unit Delay : UnitDelay  SampleTime=-1  HasFrameUpgradeWarning=on
  DeAccelTime : Outport
  wires:
  Constant2/1 -> Enabled Subsystem1/1(In1)
  Clock/1 -> Switch/3
  Unit Delay/1 -> Switch/1, DeAccelTime/1, Display/1
  Switch/1 -> Unit Delay/1
  Enable/1 -> Enabled Subsystem1/Enable
  Enabled Subsystem1/1(Out1) -> Switch/2
